simulink model "Identification"  (Simulink 7.8)
settings: Solver=FixedStepDiscrete  StartTime=0.0  StopTime=30  FixedStep=T  RelTol=1e-3
values from neighbouring files (symbols this model uses):
  NewPanto = 1    [lab_param.m]
  T = 0.001    [ABC.m]    (also in lab_param.m)
undefined symbols (not defined in the file or in its folder): HIL, qc_get_step_size
libraries: quarc_library x5
settings Model: Creator=Kjenab  LastModifiedBy=jafarm2  SimulationMode=external  ExtModeTrigDuration=100000  BufferReuse=off
settings SolverCC: PositivePriorityOrder=on
settings DataIOCC: MaxDataPoints=10000
settings OptimizationCC: BooleanDataType=off  InlineInvariantSignals=on  OptimizeBlockIOStorage=off  BufferReuse=off  ExpressionFolding=off  LocalBlockOutputs=off  InitFltsAndDblsToZero=on
settings DebuggingCC: SaveWithParameterizedLinksMsg=none  FcnCallInpInsideContextMsg=Use local settings  StrictBusMsg=Warning
settings SFSimCC: SimParseCustomCode=off
settings RTWCC: SystemTargetFile=quarc_win64.tlc  TemplateMakefile=quarc_default_tmf  Description=QUARC Win64 Target  ProcessScript=quarc_win64_make_rtw_hook
settings STFCustomTargetCC: TargetPreCompLibLocation=C:\PROGRA~3\QUARC\lib\2011b\win64\release  SystemTargetFile=quarc_win64.tlc
settings GRTTargetCC: TargetPreCompLibLocation=C:\PROGRA~3\QUARC\lib\2011b\win64\release  ParMdlRefBuildCompliant=off  CompOptLevelCompliant=off  ConcurrentExecutionCompliant=off  MatFileLogging=off  ExtMode=on  ExtModeMexFile=quarc_comm

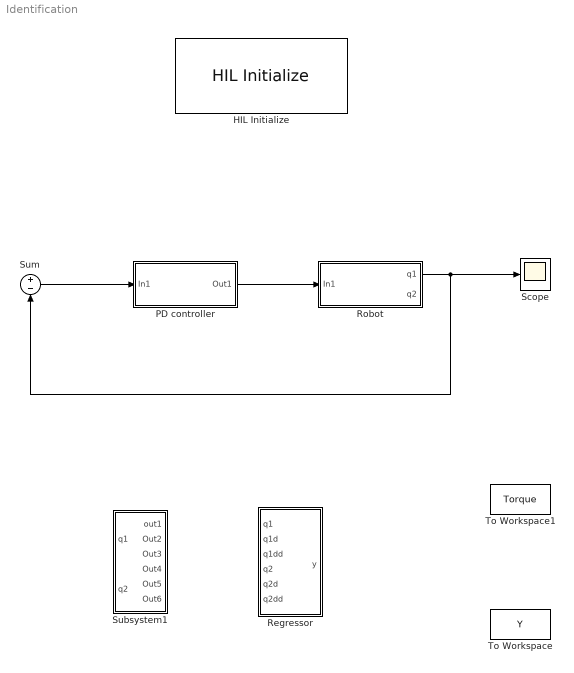
== system Identification ==
  HIL Initialize : quarc_library/Data Acquisition/Generic/Configuration/HIL Initialize  object_name=HIL-2  board_type=q4  board_number=0  exclusive=off  active=on  hardware_clocks=[0:1]  clock_modes=[0 0]  initial_clock_frequencies=[]  set_clock_params_at_start=on  set_clock_params_at_switch_in=off  set_clock_frequencies_at_start=off  set_clock_frequencies_at_switch_in=off  analog_input_channels=[0:3]  analog_input_maximums=10  analog_input_minimums=-10  set_analog_input_params_at_start=off  set_analog_input_params_at_switch_in=off  analog_output_channels=[0:3]  analog_output_maximums=[10]  analog_output_minimums=[-10]  initial_analog_outputs=[0]  final_analog_outputs=[0]  watchdog_analog_outputs=0  set_analog_output_params_at_start=on  set_analog_output_params_at_switch_in=off  set_analog_outputs_at_start=on  set_analog_outputs_at_switch_in=off  set_analog_outputs_at_terminate=on  set_analog_outputs_at_switch_out=off  set_analog_outputs_on_watchdog=off  digital_input_channels=[]  digital_output_channels=[0:3]  digital_output_configuration=[]  initial_digital_outputs=[1]  final_digital_outputs=[1]  watchdog_digital_outputs=[2]  set_digital_output_params_at_start=off  set_digital_output_params_at_switch_in=off  set_digital_outputs_at_start=on  set_digital_outputs_at_switch_in=off  set_digital_outputs_at_terminate=on  set_digital_outputs_at_switch_out=off  set_digital_outputs_on_watchdog=off  encoder_channels=[0:3]  quadrature=[4]  encoder_filter_frequency=(1/60e-9)/1  initial_encoder_counts=[0]  set_encoder_params_at_start=on  set_encoder_params_at_switch_in=off  set_encoder_counts_at_start=on  set_encoder_counts_at_switch_in=off  pwm_channels=[]  pwm_modes=[0]  pwm_frequency=(1/60e-9)/1024  pwm_configuration=[]  pwm_alignment=[]  pwm_polarity=[]  pwm_leading_deadband=[]  pwm_trailing_deadband=[]  initial_pwm_outputs=[0]  final_pwm_outputs=[0]  watchdog_pwm_outputs=[]  set_pwm_params_at_start=on  set_pwm_params_at_switch_in=off  set_pwm_outputs_at_start=on  set_pwm_outputs_at_switch_in=off  set_pwm_outputs_at_terminate=on  set_pwm_outputs_at_switch_out=off  set_pwm_outputs_on_watchdog=off  other_output_channels=[]  initial_other_outputs=[]  final_other_outputs=[]  watchdog_other_outputs=[]  set_other_outputs_at_start=off  set_other_outputs_at_switch_in=off  set_other_outputs_at_terminate=off  set_other_outputs_at_switch_out=off  set_other_outputs_on_watchdog=off
  PD controller : Subsystem
  Regressor : MATLAB Function  TreatAsAtomicUnit=on
  Robot : Subsystem
  Scope : Scope
      settings: YMin=1.05  YMax=2.1
  Subsystem1 : Subsystem
  Sum : Sum  Inputs=+-
  To Workspace : ToWorkspace  VariableName=Y  SampleTime=T  SaveFormat=Structure With Time
  To Workspace1 : ToWorkspace  VariableName=Torque  SampleTime=T  SaveFormat=Structure With Time
  wires:
  Robot/1(q1) -> Sum/2, Scope/1
  Sum/1 -> PD controller/1(In1)
  PD controller/1(Out1) -> Robot/1(In1)

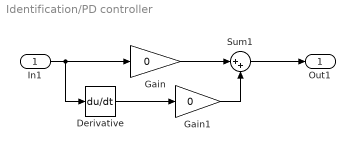
== system Identification/PD controller ==
  In1 : Inport
  Derivative : Derivative
  Gain : Gain  Gain=0
  Gain1 : Gain  Gain=0
  Sum1 : Sum  Inputs=|++
  Out1 : Outport
  wires:
  In1/1 -> Gain/1, Derivative/1
  Derivative/1 -> Gain1/1
  Gain/1 -> Sum1/1
  Sum1/1 -> Out1/1
  Gain1/1 -> Sum1/2

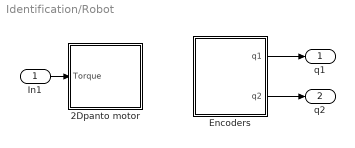
== system Identification/Robot ==
  In1 : Inport
  2Dpanto motor : Subsystem
  Encoders : Subsystem
  q1 : Outport
  q2 : Outport  Port=2
  wires:
  In1/1 -> 2Dpanto motor/1(Torque)
  Encoders/1(q1) -> q1/1
  Encoders/2(q2) -> q2/1

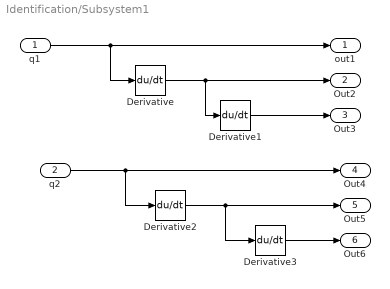
== system Identification/Subsystem1 ==
  q1 : Inport
  q2 : Inport  Port=2
  Derivative{,1..3} (4 alike) : Derivative
  out1 : Outport
  Out2 : Outport  Port=2
  Out3 : Outport  Port=3
  Out4 : Outport  Port=4
  Out5 : Outport  Port=5
  Out6 : Outport  Port=6
  wires:
  Derivative1/1 -> Out3/1
  Derivative3/1 -> Out6/1
  Derivative2/1 -> Derivative3/1, Out5/1
  q2/1 -> Derivative2/1, Out4/1
  Derivative/1 -> Derivative1/1, Out2/1
  q1/1 -> Derivative/1, out1/1

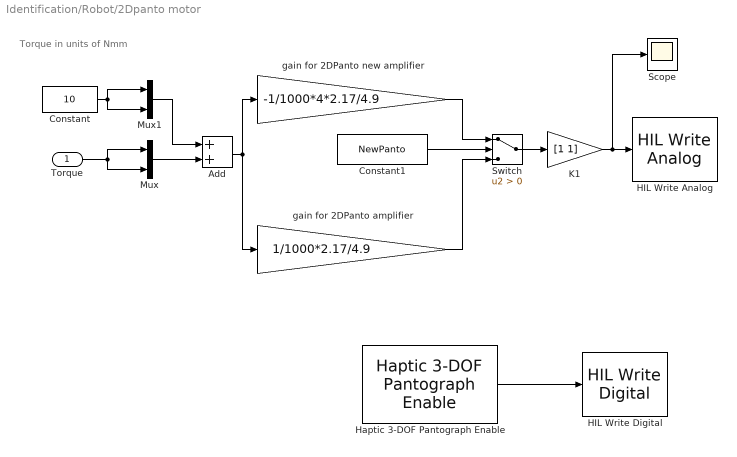
== system Identification/Robot/2Dpanto motor ==
  note: Torque in units of Nmm
  Torque : Inport
  Add : Sum
  Constant : Constant  Value=10
  Constant1 : Constant  Value=NewPanto
  HIL Write Analog : quarc_library/Data Acquisition/Generic/Immediate I//O/HIL Write Analog  object_name=HIL-2  channels=0:1  sample_time=-1  active=off  vector_input=on
  HIL Write Digital : quarc_library/Data Acquisition/Generic/Immediate I//O/HIL Write Digital  object_name=HIL-2  channels=0:3  sample_time=-1  active=off  vector_input=on
  Haptic 3-DOF Pantograph Enable : quarc_library/Devices/Quanser/Haptics/Pantographs/Haptic 3-DOF Planar Pantograph/Interfacing/Haptic 3-DOF Pantograph Enable
  K1 : Gain  Gain=[1 1]
  Mux : Mux  Inputs=2
  Mux1 : Mux  Inputs=2
  Scope : Scope
      settings: SaveName=ScopeData2
  Switch : Switch  Criteria=u2 > Threshold
  gain for 2DPanto amplifier : Gain  Gain=1/1000*2.17/4.9
  gain for 2DPanto new amplifier : Gain  Gain=-1/1000*4*2.17/4.9
  wires:
  Mux1/1 -> Add/1
  Constant/1 -> Mux1/2, Mux1/1
  Haptic 3-DOF Pantograph Enable/1 -> HIL Write Digital/1
  Mux/1 -> Add/2
  Torque/1 -> Mux/2, Mux/1
  Constant1/1 -> Switch/2
  gain for 2DPanto amplifier/1 -> Switch/3
  gain for 2DPanto new amplifier/1 -> Switch/1
  Switch/1 -> K1/1
  Add/1 -> gain for 2DPanto new amplifier/1, gain for 2DPanto amplifier/1
  K1/1 -> Scope/1, HIL Write Analog/1

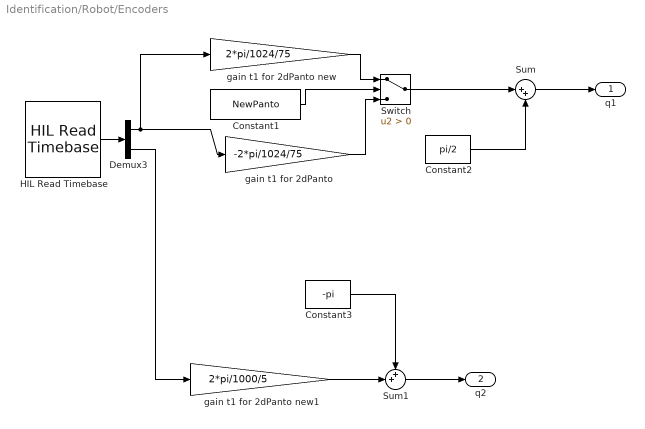
== system Identification/Robot/Encoders ==
  Constant1 : Constant  Value=NewPanto
  Constant2 : Constant  Value=pi/2
  Constant3 : Constant  Value=-pi
  Demux3 : Demux  Outputs=3
  HIL Read Timebase : quarc_library/Data Acquisition/Generic/Timebases/HIL Read Timebase  object_name=HIL-2  clock=0  analog_channels=[]  encoder_channels=[0:2]  digital_channels=[]  other_channels=[]  samples_in_buffer=max(ceil(1/qc_get_step_size), 1)  active=on  vector_output=on  data_type_mode=Inherit via back propagation  encoder_data_type=double  digital_data_type=boolean
  Sum : Sum  Inputs=|++
  Sum1 : Sum  Inputs=++|
  Switch : Switch  Criteria=u2 > Threshold
  gain t1 for 2dPanto : Gain  Gain=-2*pi/1024/75
  gain t1 for 2dPanto new : Gain  Gain=2*pi/1024/75
  gain t1 for 2dPanto new1 : Gain  Gain=2*pi/1000/5
  q1 : Outport
  q2 : Outport  Port=2
  wires:
  Sum1/1 -> q2/1
  gain t1 for 2dPanto new1/1 -> Sum1/2
  Constant3/1 -> Sum1/1
  Constant2/1 -> Sum/2
  Sum/1 -> q1/1
  Switch/1 -> Sum/1
  Demux3/3 -> gain t1 for 2dPanto new1/1
  Constant1/1 -> Switch/2
  gain t1 for 2dPanto/1 -> Switch/3
  gain t1 for 2dPanto new/1 -> Switch/1
  Demux3/1 -> gain t1 for 2dPanto new/1, gain t1 for 2dPanto/1
  HIL Read Timebase/1 -> Demux3/1

== matlab function Regressor ==
  data: q1 input double; y output double; q1d input double; q1dd input double; q2 input double; q2d input double; q2dd input double
function y = fcn(q1, q1d, q1dd, q2, q2d, q2dd)

g = 9.81;

y = zeros(2,5);
